simulink subsystem "s0326_Bad_Lyapunov"  (R2019b)
settings: Solver=VariableStepAuto  StartTime=0.0  StopTime=10.0  RelTol=1e-3
model mask{K_th=0, K_th_dot=0, K_al=0, K_al_dot=0}
undefined symbols (not defined in the file): __PRM__SERIALIZED__DATA__, PARAMS, SubsystemReferenceBlock
settings Model: Creator=francescoceresetti  LastModifiedBy=alessandro

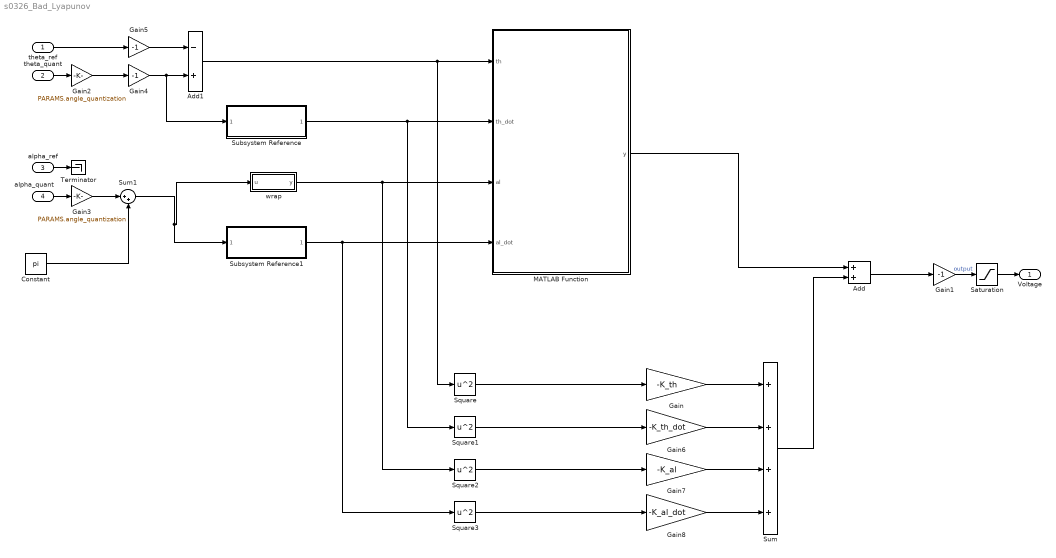
== system s0326_Bad_Lyapunov ==
  theta_ref : Inport
  theta_quant : Inport  Port=2
  alpha_ref : Inport  Port=3
  alpha_quant : Inport  Port=4
  Add : Sum
  Add1 : Sum  Inputs=-+
  Constant : Constant  Value=pi
  Gain : Gain  Gain=-K_th
  Gain1 : Gain  Gain=-1
  Gain2 : Gain  Gain=PARAMS.angle_quantization
  Gain3 : Gain  Gain=PARAMS.angle_quantization
  Gain4 : Gain  Gain=-1
  Gain5 : Gain  Gain=-1
  Gain6 : Gain  Gain=-K_th_dot
  Gain7 : Gain  Gain=-K_al
  Gain8 : Gain  Gain=-K_al_dot
  MATLAB Function : MATLAB Function  TreatAsAtomicUnit=on
  Saturation : Saturate  UpperLimit=PARAMS.V_sat  LowerLimit=-PARAMS.V_sat
  Square{,1..3} (4 alike) : Math  Operator=square  SignedPower=off  SaturateOnIntegerOverflow=on
  Subsystem Reference : Subsystem  BlockKeywords=__PRM__SERIALIZED__DATA__:SubsystemReferenceBlock  ReferencedSubsystem=Filtered_Derivative  num=num_der_filter  den=den_der_filter
  Subsystem Reference1 : Subsystem  BlockKeywords=__PRM__SERIALIZED__DATA__:SubsystemReferenceBlock  ReferencedSubsystem=Filtered_Derivative  num=num_der_filter  den=den_der_filter
  Sum : Sum  Inputs=++++
  Sum1 : Sum  Inputs=|++
  Terminator : Terminator
  wrap : MATLAB Function  TreatAsAtomicUnit=on
  Voltage : Outport
  wires:
  alpha_quant/1 -> Gain3/1
  Add1/1 -> Square/1, MATLAB Function/1(th)
  theta_quant/1 -> Gain2/1
  Subsystem Reference1/1 -> MATLAB Function/4(al_dot), Square3/1
  Subsystem Reference/1 -> MATLAB Function/2(th_dot), Square1/1
  Gain3/1 -> Sum1/1
  wrap/1(y) -> MATLAB Function/3(al), Square2/1
  Saturation/1 -> Voltage/1
  Gain4/1 -> Add1/2, Subsystem Reference/1
  Gain5/1 -> Add1/1
  theta_ref/1 -> Gain5/1
  Gain2/1 -> Gain4/1
  Gain1/1 -> Saturation/1  "output"
  alpha_ref/1 -> Terminator/1
  Add/1 -> Gain1/1
  MATLAB Function/1(y) -> Add/1
  Square/1 -> Gain/1
  Gain/1 -> Sum/1
  Square1/1 -> Gain6/1
  Gain6/1 -> Sum/2
  Square2/1 -> Gain7/1
  Gain7/1 -> Sum/3
  Square3/1 -> Gain8/1
  Gain8/1 -> Sum/4
  Sum/1 -> Add/2
  Sum1/1 -> wrap/1(u), Subsystem Reference1/1
  Constant/1 -> Sum1/2

== matlab function s0326_Bad_Lyapunov/MATLAB Function ==
  data: th input; y output; th_dot input; al input; al_dot input; PARAMS parameter
function y = fcn(th, th_dot, al, al_dot, PARAMS)
    g = PARAMS.g;

    mp = PARAMS.mp;
    Lp = PARAMS.Lp;
    mr = PARAMS.mr;
    Lr = PARAMS.Lr;
    Jm = PARAMS.Jm;

    Jh = PARAMS.Jh;
    Cal = PARAMS.Cal;
    Cth = PARAMS.Cth;

    K = PARAMS.K;
    
    R = PARAMS.Rm;
    ki = PARAMS.ki;
    kv = PARAMS.kv;



    V = -(4*Lp^4*R*mp^2*th*th_dot - 72*Cal*Jm*R*al_dot^2 - 72*Cal*Jh*R*al_dot^2 - 24*Lp^2*ki*kv*mp*th_dot^2 - 12*Cal*Lp^2*R*al_dot^2*mp - 72*Cal*Lr^2*R*al_dot^2*mp - 24*Cal*Lr^2*R*al_dot^2*mr - 24*Cth*Lp^2*R*mp*th_dot^2 + 4*Lp^4*R*al*al_dot*mp^2 - 4*Lp^4*R*al*al_dot*mp^2*cos(2*al) + 3*Lp^3*Lr*R*mp^2*th_dot^3*sin(al) - 3*Lp^3*R*al_dot*g*mp^2*sin(3*al) - 4*Lp^4*R*mp^2*th*th_dot*cos(2*al) + 3*Lp^3*Lr*R*mp^2*th_dot^3*sin(3*al) - 6*Lp^4*R*al_dot*mp^2*th_dot^2*sin(2*al) - Lp^4*R*al_dot*mp^2*th_dot^2*sin(4*al) + 15*Lp^2*Lr^2*R*al*al_dot*mp^2 + 15*Lp^2*Lr^2*R*mp^2*th*th_dot + 9*Lp^3*R*al_dot*g*mp^2*sin(al) - 9*Lp^2*Lr^2*R*al_dot^3*mp^2*sin(2*al) + 24*Jh*Lp^2*R*al*al_dot*mp + 24*Jm*Lp^2*R*al*al_dot*mp + 12*Cal*Lp^2*R*al_dot^2*mp*cos(2*al) + 24*Jh*Lp^2*R*mp*th*th_dot + 24*Jm*Lp^2*R*mp*th*th_dot - 24*K*Lp^2*R*mp*th*th_dot + 36*Lp*Lr^2*R*al_dot*g*mp^2*sin(al) + 12*Lp^2*Lr^2*R*al_dot*mp^2*th_dot^2*sin(2*al) + 36*Jh*Lp*R*al_dot*g*mp*sin(al) + 36*Jm*Lp*R*al_dot*g*mp*sin(al) + 12*Jh*Lp^2*R*al_dot*mp*th_dot^2*sin(2*al) + 12*Jm*Lp^2*R*al_dot*mp*th_dot^2*sin(2*al) - 18*Lp^3*Lr*R*al_dot^2*mp^2*th_dot*sin(al) + 9*Lp^2*Lr*R*g*mp^2*th_dot*sin(2*al) + 8*Lp^2*Lr^2*R*al*al_dot*mp*mr - 9*Lp^2*Lr^2*R*al*al_dot*mp^2*cos(2*al) + 8*Lp^2*Lr^2*R*mp*mr*th*th_dot - 6*Lp^3*Lr*R*al_dot^2*mp^2*th_dot*sin(3*al) - 9*Lp^2*Lr^2*R*mp^2*th*th_dot*cos(2*al) + 12*Lp*Lr^2*R*al_dot*g*mp*mr*sin(al) + 4*Lp^2*Lr^2*R*al_dot*mp*mr*th_dot^2*sin(2*al) - 36*Cal*Lp*Lr*R*al_dot*mp*th_dot*cos(al) - 36*Cth*Lp*Lr*R*al_dot*mp*th_dot*cos(al) - 36*K*Lp*Lr*R*al_dot*mp*th*cos(al) - 36*Lp*Lr*al_dot*ki*kv*mp*th_dot*cos(al))/(12*Lp*ki*mp*(2*Lp*th_dot + 3*Lr*al_dot*cos(al)));
    num_L = -(4*Lp^4*R*mp^2*th*th_dot - 72*Cal*Jm*R*al_dot^2 - 72*Cal*Jh*R*al_dot^2 - 24*Lp^2*ki*kv*mp*th_dot^2 - 12*Cal*Lp^2*R*al_dot^2*mp - 72*Cal*Lr^2*R*al_dot^2*mp - 24*Cal*Lr^2*R*al_dot^2*mr - 24*Cth*Lp^2*R*mp*th_dot^2 + 4*Lp^4*R*al*al_dot*mp^2 - 4*Lp^4*R*al*al_dot*mp^2*cos(2*al) + 3*Lp^3*Lr*R*mp^2*th_dot^3*sin(al) - 3*Lp^3*R*al_dot*g*mp^2*sin(3*al) - 4*Lp^4*R*mp^2*th*th_dot*cos(2*al) + 3*Lp^3*Lr*R*mp^2*th_dot^3*sin(3*al) - 6*Lp^4*R*al_dot*mp^2*th_dot^2*sin(2*al) - Lp^4*R*al_dot*mp^2*th_dot^2*sin(4*al) + 15*Lp^2*Lr^2*R*al*al_dot*mp^2 + 15*Lp^2*Lr^2*R*mp^2*th*th_dot + 9*Lp^3*R*al_dot*g*mp^2*sin(al) - 9*Lp^2*Lr^2*R*al_dot^3*mp^2*sin(2*al) + 24*Jh*Lp^2*R*al*al_dot*mp + 24*Jm*Lp^2*R*al*al_dot*mp + 12*Cal*Lp^2*R*al_dot^2*mp*cos(2*al) + 24*Jh*Lp^2*R*mp*th*th_dot + 24*Jm*Lp^2*R*mp*th*th_dot - 24*K*Lp^2*R*mp*th*th_dot + 36*Lp*Lr^2*R*al_dot*g*mp^2*sin(al) + 12*Lp^2*Lr^2*R*al_dot*mp^2*th_dot^2*sin(2*al) + 36*Jh*Lp*R*al_dot*g*mp*sin(al) + 36*Jm*Lp*R*al_dot*g*mp*sin(al) + 12*Jh*Lp^2*R*al_dot*mp*th_dot^2*sin(2*al) + 12*Jm*Lp^2*R*al_dot*mp*th_dot^2*sin(2*al) - 18*Lp^3*Lr*R*al_dot^2*mp^2*th_dot*sin(al) + 9*Lp^2*Lr*R*g*mp^2*th_dot*sin(2*al) + 8*Lp^2*Lr^2*R*al*al_dot*mp*mr - 9*Lp^2*Lr^2*R*al*al_dot*mp^2*cos(2*al) + 8*Lp^2*Lr^2*R*mp*mr*th*th_dot - 6*Lp^3*Lr*R*al_dot^2*mp^2*th_dot*sin(3*al) - 9*Lp^2*Lr^2*R*mp^2*th*th_dot*cos(2*al) + 12*Lp*Lr^2*R*al_dot*g*mp*mr*sin(al) + 4*Lp^2*Lr^2*R*al_dot*mp*mr*th_dot^2*sin(2*al) - 36*Cal*Lp*Lr*R*al_dot*mp*th_dot*cos(al) - 36*Cth*Lp*Lr*R*al_dot*mp*th_dot*cos(al) - 36*K*Lp*Lr*R*al_dot*mp*th*cos(al) - 36*Lp*Lr*al_dot*ki*kv*mp*th_dot*cos(al));
    den_L = (12*Lp*ki*mp*(2*Lp*th_dot + 3*Lr*al_dot*cos(al)));
    
    if den_L == 0 && num_L == 0
        V = 0.02;
    else 
        V = num_L/den_L;
    end
    
    
y = V;

== matlab function s0326_Bad_Lyapunov/wrap ==
  data: u input; y output
function y = wrap(u)
stop_condition = false;
y = u;
while ~stop_condition
    if y > pi
        y = y - 2*pi;
    elseif y < -pi
        y = y + 2*pi;
    else
        stop_condition = true;
    end
end
